simulink model "valva"  (R2022b)
settings: Solver=ode3  StartTime=0.0  StopTime=2  FixedStep=0.001  RelTol=1e-3
settings Model: Creator=rus_d  LastModifiedBy=rus_d
settings SolverCC: ZeroCrossAlgorithm=Adaptive
settings DataIOCC: ReturnWorkspaceOutputs=off
settings DebuggingCC: IgnoredZcDiagnostic=none

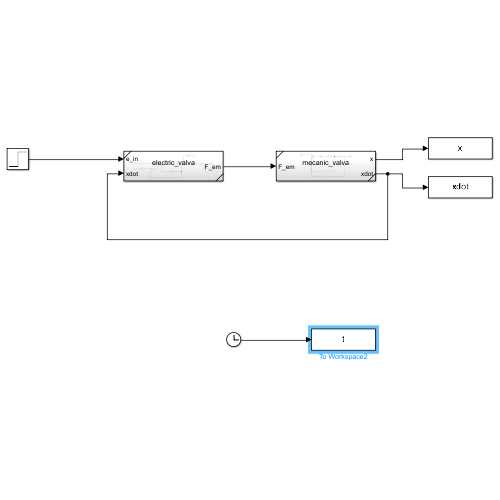
[thumbnail: Simulink's stored preview of the top-level diagram]
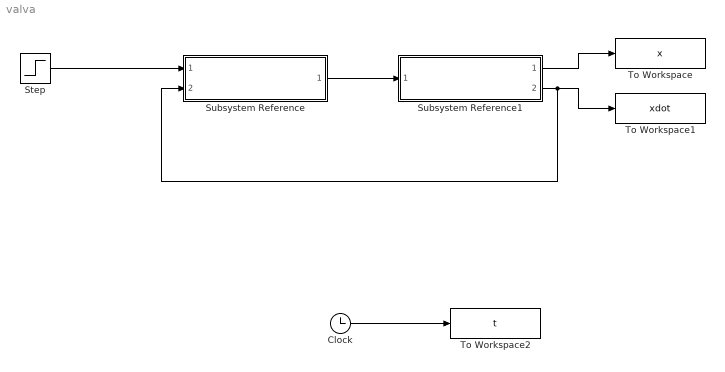
== system valva ==
  Clock : Clock
  Step : Step  Time=0.05  After=10  SampleTime=0
  Subsystem Reference : Subsystem  ReferencedSubsystem=electric_valva
  Subsystem Reference1 : Subsystem  ReferencedSubsystem=mecanic_valva
  To Workspace : ToWorkspace  VariableName=x  SampleTime=-1
  To Workspace1 : ToWorkspace  VariableName=xdot  SampleTime=-1
  To Workspace2 : ToWorkspace  VariableName=t  SampleTime=-1
  wires:
  Step/1 -> Subsystem Reference/1
  Subsystem Reference/1 -> Subsystem Reference1/1
  Subsystem Reference1/1 -> To Workspace/1
  Subsystem Reference1/2 -> Subsystem Reference/2, To Workspace1/1
  Clock/1 -> To Workspace2/1
